simulink model "final_fifth_order_plan"  (R2020a)
settings: Solver=VariableStepAuto  StartTime=0.0  StopTime=inf  RelTol=1e-3
libraries: simulink x1
settings Model: EnablePacing=on  Creator=nose  LastModifiedBy=nose

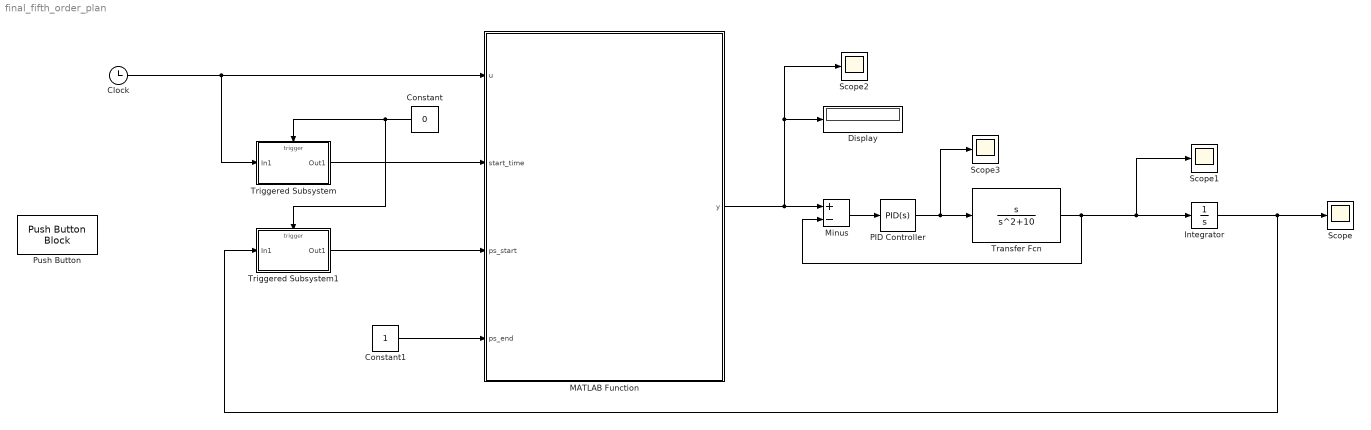
== system final_fifth_order_plan ==
  Clock : Clock
  Constant : Constant  Value=0
  Constant1 : Constant
  Display : Display
  Integrator : Integrator
  MATLAB Function : MATLAB Function  TreatAsAtomicUnit=on
  Minus : Sum  Inputs=+-
  PID Controller : simulink/Continuous/PID Controller  Controller=PID  Form=Parallel  TimeDomain=Continuous-time  UseExternalTs=off  SampleTime=-1  IntegratorMethod=Forward Euler  FilterMethod=Forward Euler  ControllerParametersSource=internal  P=91.031435379878  I=1537.46891029959  D=-0.0368135406568258  UseFilter=on  N=91.3566495233405  TunerSelectOption=Transfer Function Based (PID Tuner App)  InitialConditionSource=internal  InitialConditionForIntegrator=0  InitialConditionForFilter=0  DifferentiatorICPrevScaledInput=0  ExternalReset=none  TrackingMode=off  Kt=1  LimitOutput=off  UpperSaturationLimit=inf  LowerSaturationLimit=-inf  LinearizeAsGain=on  AntiWindupMode=none  Kb=1  POutMin=[]  POutMax=[]  IOutMin=[]  IOutMax=[]  DOutMin=[]  DOutMax=[]  NOutMin=[]  NOutMax=[]  SumOutMin=[]  SumOutMax=[]  SaturationOutMin=[]  SaturationOutMax=[]  PParamMin=[]  PParamMax=[]  IParamMin=[]  IParamMax=[]  DParamMin=[]  DParamMax=[]  NParamMin=[]  NParamMax=[]  KbParamMin=[]  KbParamMax=[]  KtParamMin=[]  KtParamMax=[]  KbOutMin=[]  KbOutMax=[]  KtOutMin=[]  KtOutMax=[]  IntegratorOutMin=[]  IntegratorOutMax=[]  FilterOutMin=[]  FilterOutMax=[]  SumI1OutMin=[]  SumI1OutMax=[]  SumI2OutMin=[]  SumI2OutMax=[]  SumI3OutMin=[]  SumI3OutMax=[]  SumI4OutMin=[]  SumI4OutMax=[]  SumDOutMin=[]  SumDOutMax=[]  DifferentiatorOutMin=[]  DifferentiatorOutMax=[]  FilterDiffOutCoefMin=[]  FilterDiffOutCoefMax=[]  ReciprocalOutMin=[]  ReciprocalOutMax=[]  SumDenOutMin=[]  SumDenOutMax=[]  SumNumOutMin=[]  SumNumOutMax=[]  DivideOutMin=[]  DivideOutMax=[]  UdiffTsProdOutMin=[]  UdiffTsProdOutMax=[]  NTsProdOutMin=[]  NTsProdOutMax=[]  UintegralTsProdOutMin=[]  UintegralTsProdOutMax=[]  UngainTsProdOutMin=[]  UngainTsProdOutMax=[]  IntegratorContinuousStateAttributes=''  IntegratorStateMustResolveToSignalObject=off  IntegratorRTWStateStorageClass=Auto  FilterContinuousStateAttributes=''  FilterStateMustResolveToSignalObject=off  FilterRTWStateStorageClass=Auto  ParallelPVariant=InternalParameters  IdealPVariant=Disabled  IVariant=InternalParameters  DVariant=InternalParameters  IntegratorVariant=Continuous  SatVariant=Disabled  AWVariant=Passthrough  PCopyVariant=Disabled  TRVariant=Disabled  FdbkBlocksVariant=Forward  IdealPFdbkVariant=Disabled  SatFdbkVariant=Disabled  DerivativeFilterVariant=ContFilter  NVariant=InternalParameters  NCopyVariant=Disabled  FilterICVariant=InternalICsFilter  IntegratorICVariant=InternalICs  ExternalResetVariant=Disabled  TRSumVariant=Passthrough  SumFdbkVariant=Disabled  SumVariant=Sum_PID  TsampFilterVariant=InternalTs  TsampNgainVariant=Passthrough  TsampIntegralVariant=Passthrough
  Push Button : PushButtonBlock
  Scope{,1..3} (4 alike) : Scope
  Transfer Fcn : TransferFcn  Numerator=[1 0]  Denominator=[1 0 10]
  Triggered Subsystem : Subsystem  TreatAsAtomicUnit=on
  Triggered Subsystem1 : Subsystem  TreatAsAtomicUnit=on
  wires:
  PID Controller/1 -> Scope3/1, Transfer Fcn/1
  Minus/1 -> PID Controller/1
  Transfer Fcn/1 -> Scope1/1, Integrator/1, Minus/2
  MATLAB Function/1(y) -> Scope2/1, Display/1, Minus/1
  Triggered Subsystem1/1(Out1) -> MATLAB Function/3(ps_start)
  Triggered Subsystem/1(Out1) -> MATLAB Function/2(start_time)
  Clock/1 -> Triggered Subsystem/1(In1), MATLAB Function/1(u)
  Integrator/1 -> Triggered Subsystem1/1(In1), Scope/1
  Constant1/1 -> MATLAB Function/4(ps_end)
  Constant/1 -> Triggered Subsystem1/Trigger, Triggered Subsystem/Trigger

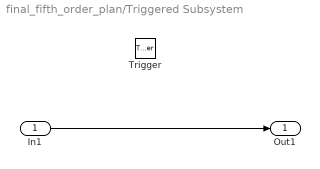
== system final_fifth_order_plan/Triggered Subsystem ==
  In1 : Inport
  Trigger : TriggerPort  VariantControl=Variant
  Out1 : Outport
  wires:
  In1/1 -> Out1/1

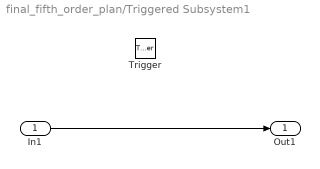
== system final_fifth_order_plan/Triggered Subsystem1 ==
  In1 : Inport
  Trigger : TriggerPort  VariantControl=Variant
  Out1 : Outport
  wires:
  In1/1 -> Out1/1

== matlab function final_fifth_order_plan/MATLAB Function ==
  data: u input; y output; start_time input; ps_start input; ps_end input
function y = fcn(u,start_time,ps_start,ps_end)
out = 0;
%ps_start = -pi
%ps_end = pi
inverse = 0;
dis = ps_end - ps_start;
if dis < 0
    inverse = 1;
    dis = dis*-1;
end
ps_start = 0;
ps_end = dis;


Vmax= 1.5;
amax = 12;
tf = 15*(ps_end-ps_start)/(8*Vmax)
%tf = ((45*ps_end-ps_start)/(2*amax))^(1/2)/2
%tf = ((23*ps_end-ps_start)/(amax))^(1/2)/2;
t = (0:0.01:tf)';
a0 = ps_start;
a1 = 0;
a2 = 0;
a3 = 10*(ps_end-ps_start)/(tf^3);
a4 = -15*(ps_end-ps_start)/(tf^4);
a5 = 6*(ps_end-ps_start)/(tf^5);


w = @(t) a1+2.*a2.*t + 3.*a3.*t.^2 + 4.*a4.*t.^3 + 5.*a5.*t.^4;
velocity = w(t);

if inverse
    velocity = velocity*-1;
end

if floor((u-start_time) / 0.01) + 1 < size(t,1)
    if(floor((u-start_time) / 0.01) + 1 <=0)
        out = velocity(1);
    else
        out = velocity (floor((u-start_time) / 0.01) + 1);
    end
end



y = out;
